simulink model "hw3_compare_in_simulink"  (R2021b)
settings: Solver=VariableStepAuto  StartTime=0.0  StopTime=10.0  RelTol=1e-3
values from neighbouring files (symbols this model uses):
  Fm = 0.00001*r^2    (= 1e-05)    [hw3.m]
  Im = 0.0003*r^2    (= 0.0003)    [hw3.m]
  Kt = 0.0705*r    (= 0.0705)    [hw3.m]
  La = 0.000264    [hw3.m]
  Ra = 0.343    [hw3.m]
settings Model: Creator=86180  LastModifiedBy=86180

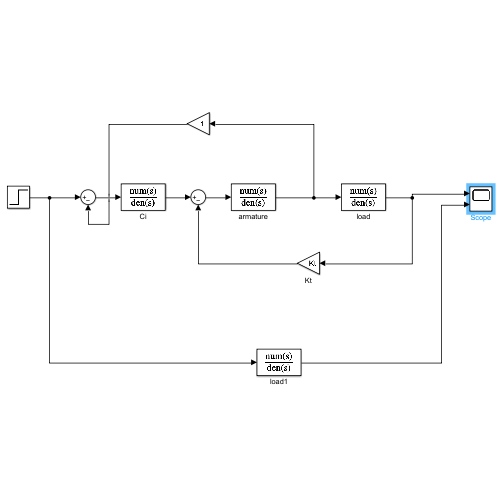
[thumbnail: Simulink's stored preview of the top-level diagram]
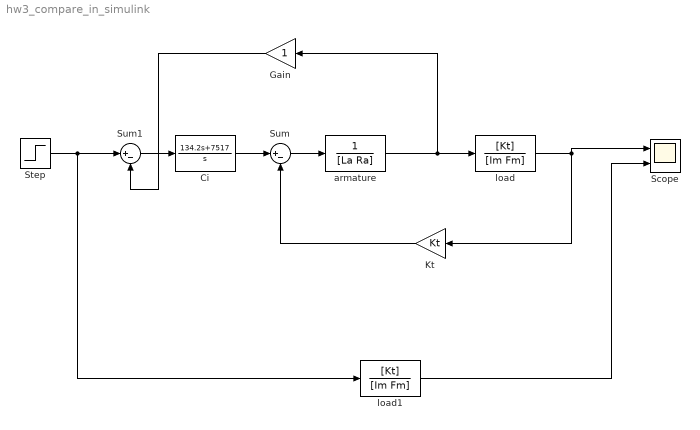
== system hw3_compare_in_simulink ==
  Ci : TransferFcn  Numerator=[134.2 7517]  Denominator=[1 0]
  Gain : Gain
  Kt : Gain  Gain=Kt
  Scope : Scope  NumInputPorts=2
  Step : Step  SampleTime=0
  Sum : Sum  Inputs=|+-
  Sum1 : Sum  Inputs=|+-
  armature : TransferFcn  Denominator=[La Ra]
  load : TransferFcn  Numerator=[Kt]  Denominator=[Im Fm]
  load1 : TransferFcn  Numerator=[Kt]  Denominator=[Im Fm]
  wires:
  Ci/1 -> Sum/1
  Sum/1 -> armature/1
  Kt/1 -> Sum/2
  load/1 -> Scope/1, Kt/1
  armature/1 -> Gain/1, load/1
  Sum1/1 -> Ci/1
  Gain/1 -> Sum1/2
  Step/1 -> load1/1, Sum1/1
  load1/1 -> Scope/2
